simulink model "L4_simulink"  (R2024b)
settings: Solver=VariableStepAuto  StartTime=0.0  StopTime=10.0  RelTol=1e-3
undefined symbols (not defined in the file or in its folder): K1, K2, T
settings Model: Creator=syaba  LastModifiedBy=Salvador

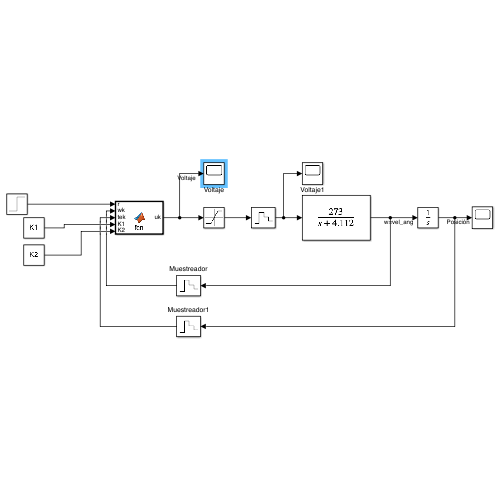
[thumbnail: Simulink's stored preview of the top-level diagram]
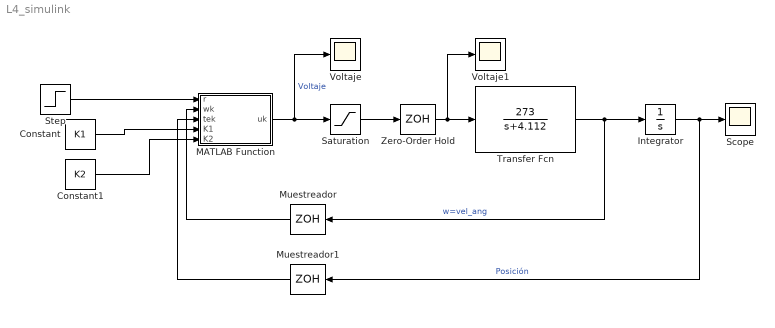
== system L4_simulink ==
  Constant : Constant  Value=K1
  Constant1 : Constant  Value=K2  VectorParams1D=off
  Integrator : Integrator
  MATLAB Function : MATLAB Function  TreatAsAtomicUnit=on  SystemSampleTime=T
  Muestreador : ZeroOrderHold  SampleTime=T
  Muestreador1 : ZeroOrderHold  SampleTime=T
  Saturation : Saturate  UpperLimit=3  LowerLimit=-3
  Scope : Scope
  Step : Step  Time=0  After=100  SampleTime=0
  Transfer Fcn : TransferFcn  Numerator=[273]  Denominator=[1 4.112]
  Voltaje : Scope
  Voltaje1 : Scope
  Zero-Order Hold : ZeroOrderHold  SampleTime=T
  wires:
  Transfer Fcn/1 -> Muestreador/1, Integrator/1  "w=vel_ang"
  MATLAB Function/1(uk) -> Voltaje/1, Saturation/1  "Voltaje"
  Zero-Order Hold/1 -> Voltaje1/1, Transfer Fcn/1
  Integrator/1 -> Scope/1, Muestreador1/1  "Posición"
  Constant/1 -> MATLAB Function/4(K1)
  Constant1/1 -> MATLAB Function/5(K2)
  Step/1 -> MATLAB Function/1(r)
  Muestreador/1 -> MATLAB Function/2(wk)
  Muestreador1/1 -> MATLAB Function/3(tek)
  Saturation/1 -> Zero-Order Hold/1

== matlab function L4_simulink/MATLAB Function ==
  data: r input; uk output; wk input; tek input; K1 input; K2 input
function uk = fcn(r, wk, tek, K1, K2)

persistent vk_1;

if isempty(vk_1)
    vk_1 = 0
end;

xk = [tek
      wk];

ek = r-tek;
vk = vk_1 + ek;
uk = K1*vk - K2*xk;

vk_1 = vk;
